simulink model "SegheriaSCADA2"  (R2024b)
settings: Solver=FixedStepAuto  StartTime=0.0  StopTime=2000  FixedStep=0.025  RelTol=1e-3
values from neighbouring files (symbols this model uses):
  b = t + 2*s    (= 3.6)    [ParametriSegheria.m]    (also in ParametriSegheriaDinamica.m; main_param_CLASSIC.m; main_param_SCADA.m)
  b2 = t2 + 2*s2    (= 10)    [ParametriSegheria.m]    (also in ParametriSegheriaDinamica.m; main_param_CLASSIC.m; main_param_SCADA.m)
  h_index = [70, 80, 90, 100]    [ParametriSegheria.m]    (also in ParametriSegheriaDinamica.m = [80, 90, 100]; main_param_CLASSIC.m = [80, 90, 100, 110]; main_param_SCADA.m = [80, 90, 100, 110])
  h_start_1 = 1    [main_param_CLASSIC.m]
  h_start_2 = 2    [main_param_CLASSIC.m]
  h_start_3 = 3    [main_param_CLASSIC.m]
  h_start_4 = 1    [main_param_CLASSIC.m]
  h_start_5 = 2    [main_param_CLASSIC.m]
  h_start_6 = 3    [main_param_CLASSIC.m]
  i_id = 60    [ParametriSegheria.m]
  i_id2 = 60    [ParametriSegheria.m]
  i_max = 100    [ParametriSegheria.m]
  kc = [0 35 40 50 55 90]    [ParametriSegheria.m]    (also in ParametriSegheriaDinamica.m = [0, 25, 30, 35, 50, 70]; main_param_CLASSIC.m = [0, 25, 30, 35, 50, 70]; main_param_SCADA.m = [0, 25, 30, 35, 50, 70])
  Kt = 2    [ParametriSegheria.m]    (also in ParametriSegheriaDinamica.m = 10000; main_param_CLASSIC.m = 10000; main_param_SCADA.m = 10000)
  Kt2 = 5    [ParametriSegheria.m]    (also in ParametriSegheriaDinamica.m = 4500; main_param_CLASSIC.m = 4500; main_param_SCADA.m = 4500)
  l_index = [20, 30, 40, 50]    [ParametriSegheria.m]    (also in ParametriSegheriaDinamica.m = [30, 40, 50]; main_param_CLASSIC.m = [30, 40, 50, 60]; main_param_SCADA.m = [30, 40, 50, 60])
  l_start_1 = 1    [main_param_CLASSIC.m]
  l_start_2 = 1    [main_param_CLASSIC.m]
  l_start_3 = 1    [main_param_CLASSIC.m]
  l_start_4 = 1    [main_param_CLASSIC.m]
  l_start_5 = 1    [main_param_CLASSIC.m]
  l_start_6 = 1    [main_param_CLASSIC.m]
  Lt = 4    [ParametriSegheria.m]    (also in ParametriSegheriaDinamica.m; main_param_CLASSIC.m; main_param_SCADA.m)
  Mag_D1 = [0 randi([220 500], 1, 40)]    [ParametriSegheria.m]    (also in ParametriSegheriaDinamica.m = [0 randi([200 500], 1, N_log)]; main_param_CLASSIC.m = [0 randi([200 500], 1, N_log)]; main_param_SCADA.m = [0 randi([200 500], 1, N_log)])
  Mag_D2 = [0 randi([220 500], 1, 40)]    [ParametriSegheria.m]    (also in ParametriSegheriaDinamica.m = [0 randi([200 500], 1, N_log)]; main_param_CLASSIC.m = [0 randi([200 500], 1, N_log)]; main_param_SCADA.m = [0 randi([200 500], 1, N_log)])
  Mag_D3 = [0 randi([220 500], 1, 40)]    [ParametriSegheria.m]    (also in ParametriSegheriaDinamica.m = [0 randi([200 500], 1, N_log)]; main_param_CLASSIC.m = [0 randi([200 500], 1, N_log)]; main_param_SCADA.m = [0 randi([200 500], 1, N_log)])
  Mag_legno1 = [0 randi([1 5], 1, 40)]    [ParametriSegheria.m]    (also in ParametriSegheriaDinamica.m = [0 randi([1 5], 1, N_log)]; main_param_CLASSIC.m = [0 randi([1 5], 1, N_log)]; main_param_SCADA.m = [0 randi([1 5], 1, N_log)])
  Mag_legno2 = [0 randi([1 5], 1, 40)]    [ParametriSegheria.m]    (also in ParametriSegheriaDinamica.m = [0 randi([1 5], 1, N_log)]; main_param_CLASSIC.m = [0 randi([1 5], 1, N_log)]; main_param_SCADA.m = [0 randi([1 5], 1, N_log)])
  Mag_legno3 = [0 randi([1 5], 1, 40)]    [ParametriSegheria.m]    (also in ParametriSegheriaDinamica.m = [0 randi([1 5], 1, N_log)]; main_param_CLASSIC.m = [0 randi([1 5], 1, N_log)]; main_param_SCADA.m = [0 randi([1 5], 1, N_log)])
  n_sottili = 4    [ParametriSegheria.m]
  omega = 50    [ParametriSegheria.m]
  omega2 = 3000*(2*pi/60)    (= 314.159265359)    [ParametriSegheria.m]
  SR = Rs/Rm    (= 5.33333333333)    [ParametriSegheria.m]    (also in ParametriSegheriaDinamica.m; main_param_CLASSIC.m; main_param_SCADA.m)
  SR2 = Rc/Rm2    (= 4)    [ParametriSegheria.m]    (also in ParametriSegheriaDinamica.m; main_param_CLASSIC.m; main_param_SCADA.m)
  thrsh = 40    [ParametriSegheria.m]
  Tloss = Tatt+ Tdamp    (= 17.3333333333)    [ParametriSegheria.m]
  Tloss2 = Tatt2+ Tdamp2    (= 66.8318530718)    [ParametriSegheria.m]
libraries: simulink x15, slpidlib x9
(part 3 of 3)

== matlab function SegheriaSCADA2/Linea 2/Macchina 2/MATLAB Function2 ==
  settings: updateMethod=DISCRETE
  data: u input; w_asse input; y output; l_asse input; taglio output; Lt parameter
function [y, taglio] = fcn(u, w_asse, l_asse,Lt)
    persistent counter 

    n_assi = floor(l_asse / w_asse);
    
    taglio = 0;

    if isempty(counter)
        counter = 0;
    end

    % Conto assi tagliate
    if u >= Lt
        counter = counter + n_assi;
    end

    % Segnale di taglio
    if  (u > 0 && u < Lt && l_asse > 0) 
        taglio = 1;
    end

    y = counter;
end

== matlab function SegheriaSCADA2/Linea 2/Macchina 3/MATLAB Function2 ==
  settings: updateMethod=DISCRETE
  data: u input; w_asse input; y output; l_asse input; taglio output; Lt parameter
function [y, taglio] = fcn(u, w_asse, l_asse,Lt)
    persistent counter 

    n_assi = floor(l_asse / w_asse);
    
    taglio = 0;

    if isempty(counter)
        counter = 0;
    end

    % Conto assi tagliate
    if u >= Lt
        counter = counter + n_assi;
    end

    % Segnale di taglio
    if  (u > 0 && u < Lt && l_asse > 0) 
        taglio = 1;
    end

    y = counter;
end

== matlab function SegheriaSCADA2/Linea 3/MATLAB Function ==
  data: u input; y output
function y = fcn(u)

    persistent n_prec

    if isempty(n_prec)
        n_prec = 0;
    end

    y = u - n_prec;


    n_prec = u;

== matlab function SegheriaSCADA2/Linea 3/MATLAB Function1 ==
  data: u input; y output
function y = fcn(u)

    persistent n_prec

    if isempty(n_prec)
        n_prec = 0;
    end

    y = u - n_prec;

    n_prec = u;

== matlab function SegheriaSCADA2/Linea 3/Macchina 1/Logica Macchina 1/MATLAB Function ==
  data: u input; y output; Mag_legno3 parameter
function y = fcn(u, Mag_legno3)
    persistent counter
    if isempty(counter)
        counter = 1;
    end

    if u == 1
        counter = counter + 1;
    end

    y = counter;
    
    if y > length(Mag_legno3)-1
        y = 0;
    end

end

== matlab function SegheriaSCADA2/Linea 3/Macchina 1/Logica Macchina 1/MATLAB Function2 ==
  settings: updateMethod=DISCRETE
  data: spessore input; u input; spessore2 input; thin_cut input; diametro input; y output; larg_asse output; thickness output; finito output
function [y, larg_asse, thickness, finito]= fcn(spessore, u, spessore2, thin_cut, diametro)
    persistent counter 

  
    max_assi = floor((diametro-thin_cut*spessore2) / spessore);
    finito = 0;
    
    if isempty(counter)
        counter = 0;
    end

    % Conto assi tagliate
    if u == 1
        counter = counter + 1;
    end

    % Quando finisco tronco segnalo e azzero counter
    if counter > max_assi + thin_cut
        finito = 1;
        counter = 0;
    end

    
    if counter == 0
        larg_asse = 0;
        thickness = 0;
    elseif counter <= thin_cut/2
        distanza_bordo = counter * spessore2;
        h = abs(diametro/2 - distanza_bordo + (spessore2/2));
        larg_asse = 2 * sqrt((diametro/2)^2-h^2);
        thickness = spessore2;
    elseif counter > max_assi + thin_cut/2
        distanza_bordo = max_assi*spessore + (counter-max_assi)*spessore2;
        h = abs(diametro/2 - distanza_bordo + (spessore2/2));
        larg_asse = 2 * sqrt((diametro/2)^2-h^2);
        thickness = spessore2;
    else
        % Calcolo larghezza delle assi
        distanza_bordo = thin_cut/2 * spessore2 + (counter-thin_cut/2) * spessore;
        h = abs(diametro/2 - distanza_bordo + (spessore/2));
        larg_asse = 2 * sqrt((diametro/2)^2-h^2);
        thickness = spessore;
    end
    

    y = counter;

== matlab function SegheriaSCADA2/Linea 1/Macchina 2/MATLAB Function2 ==
  settings: updateMethod=DISCRETE
  data: u input; w_asse input; y output; l_asse input; taglio output; Lt parameter
function [y, taglio] = fcn(u, w_asse, l_asse,Lt)
    persistent counter 

    n_assi = floor(l_asse / w_asse);
    
    taglio = 0;

    if isempty(counter)
        counter = 0;
    end

    % Conto assi tagliate
    if u >= Lt
        counter = counter + n_assi;
    end

    % Segnale di taglio
    if  (u > 0 && u < Lt && l_asse > 0) 
        taglio = 1;
    end

    y = counter;
end

== matlab function SegheriaSCADA2/Linea 3/Macchina 2/MATLAB Function2 ==
  settings: updateMethod=DISCRETE
  data: u input; w_asse input; y output; l_asse input; taglio output; Lt parameter
function [y, taglio] = fcn(u, w_asse, l_asse,Lt)
    persistent counter 

    n_assi = floor(l_asse / w_asse);
    
    taglio = 0;

    if isempty(counter)
        counter = 0;
    end

    % Conto assi tagliate
    if u >= Lt
        counter = counter + n_assi;
    end

    % Segnale di taglio
    if  (u > 0 && u < Lt && l_asse > 0) 
        taglio = 1;
    end

    y = counter;
end

== matlab function SegheriaSCADA2/Linea 3/Macchina 3/MATLAB Function2 ==
  settings: updateMethod=DISCRETE
  data: u input; w_asse input; y output; l_asse input; taglio output; Lt parameter
function [y, taglio] = fcn(u, w_asse, l_asse,Lt)
    persistent counter 

    n_assi = floor(l_asse / w_asse);
    
    taglio = 0;

    if isempty(counter)
        counter = 0;
    end

    % Conto assi tagliate
    if u >= Lt
        counter = counter + n_assi;
    end

    % Segnale di taglio
    if  (u > 0 && u < Lt && l_asse > 0) 
        taglio = 1;
    end

    y = counter;
end

== matlab function SegheriaSCADA2/Subsystem1/MATLAB Function6 ==
  data: u input; idx output; h_index parameter
function idx = find_index(u, h_index)
%#codegen

v = h_index;

idx = -1; % valore default se non trovato

for i = 1:length(v)
    if u == v(i)
        idx = i;
        return;
    end
end

== matlab function SegheriaSCADA2/Subsystem1/MATLAB Function7 ==
  data: u input; idx output; h_index parameter
function idx = find_index(u, h_index)
%#codegen

v = h_index;

idx = -1; % valore default se non trovato

for i = 1:length(v)
    if u == v(i)
        idx = i;
        return;
    end
end

== matlab function SegheriaSCADA2/Subsystem1/MATLAB Function8 ==
  data: u input; idx output; h_index parameter
function idx = find_index(u, h_index)
%#codegen

v = h_index;

idx = -1; % valore default se non trovato

for i = 1:length(v)
    if u == v(i)
        idx = i;
        return;
    end
end

== matlab function SegheriaSCADA2/Subsystem1/MATLAB Function9 ==
  data: u input; idx output; h_index parameter
function idx = find_index(u, h_index)
%#codegen

v = h_index;

idx = -1; % valore default se non trovato

for i = 1:length(v)
    if u == v(i)
        idx = i;
        return;
    end
end

== matlab function SegheriaSCADA2/Subsystem1/MATLAB Function10 ==
  data: u input; idx output; l_index parameter
function idx = find_index(u, l_index)
%#codegen

v = l_index;

idx = -1; % valore default se non trovato

for i = 1:length(v)
    if u == v(i)
        idx = i;
        return;
    end
end

== matlab function SegheriaSCADA2/Subsystem1/MATLAB Function11 ==
  data: u input; idx output; l_index parameter
function idx = find_index(u, l_index)
%#codegen

v = l_index;

idx = -1; % valore default se non trovato

for i = 1:length(v)
    if u == v(i)
        idx = i;
        return;
    end
end

== matlab function SegheriaSCADA2/Subsystem1/MATLAB Function12 ==
  data: u input; idx output; l_index parameter
function idx = find_index(u, l_index)
%#codegen

v = l_index;

idx = -1; % valore default se non trovato

for i = 1:length(v)
    if u == v(i)
        idx = i;
        return;
    end
end

== matlab function SegheriaSCADA2/Subsystem1/MATLAB Function13 ==
  data: u input; idx output; l_index parameter
function idx = find_index(u, l_index)
%#codegen

v = l_index;

idx = -1; % valore default se non trovato

for i = 1:length(v)
    if u == v(i)
        idx = i;
        return;
    end
end

== matlab function SegheriaSCADA2/Subsystem1/MATLAB Function14 ==
  data: h_next output; Magazzino output; work output; l_next output; h_idx input; target_matrice parameter; n_assi input; l_idx input
function [h_next, Magazzino, work, l_next] = fcn(h_idx, target_matrice, n_assi, l_idx)

[n_rows, n_cols] = size(target_matrice);

h_next = zeros(1,length(h_idx));
l_next = zeros(1,length(l_idx));

persistent MagazzinoGlobale

for i = 1:length(n_assi)

    if isempty(MagazzinoGlobale)
        MagazzinoGlobale = zeros(n_rows, n_cols);
    end


    % Output iniziali
    h_next(i) = h_idx(i);
    l_next(i) = l_idx(i);


    MagazzinoGlobale(h_idx(i), l_idx(i)) = MagazzinoGlobale(h_idx(i), l_idx(i)) + n_assi(i);

    work = 1;

    if MagazzinoGlobale(h_idx(i), l_idx(i)) >= target_matrice(h_idx(i), l_idx(i))


        deficit = target_matrice - MagazzinoGlobale;

        best_cost = inf;
        best_h = h_idx(i);
        best_l = l_idx(i);

        for h = 1:n_rows
            for l = 1:n_cols

                if deficit(h,l) > 0

                    % Penalità cambio lama
                    cambio = (l ~= l_idx(i));

                    % Funzione costo
                    cost = -deficit(h,l) + 60*cambio;

                    if cost < best_cost
                        best_cost = cost;
                        best_h = h;
                        best_l = l;
                    end
                end

            end
        end

        if best_cost < inf
            h_next(i) = best_h;
            l_next(i) = best_l;
        else
            work = 0;
        end

    end
end

Magazzino = MagazzinoGlobale;

== matlab function SegheriaSCADA2/Linea 1/Macchina 1/Dinamica Macchina 1/MATLAB Function ==
  settings: updateMethod=DISCRETE
  data: u input; y output; t input
function y = f(u, t)
persistent t_start active

if isempty(active)
    active = false;
    t_start = 0;
end

if u == 1 && ~active
    t_start = t;
    active = true;
end

if active
    if (t - t_start) <= 180
        y = 0;
    else
        y = 1;
        active = false;
    end
else
    y = 1;
end

== matlab function SegheriaSCADA2/Subsystem1/CAMBIO LAME CONSUMATE ==
  data: n_assi input; y output; cambio_1 output; cambio_2 output; cambio_3 output
function [y, cambio_1, cambio_2, cambio_3] = fcn(n_assi)

    warning = zeros(1, length(n_assi));

    persistent usura_lama

    if isempty(usura_lama)
        usura_lama = zeros(1, length(n_assi));
    end

    cambio_1 = 0;
    cambio_2 = 0;
    cambio_3 = 0;

    for i = 1:length(n_assi)
        
        % Ogni volta che arriva un certo numero di assi vuol dire che le
        % lame hanno appena fatto un taglio
        if n_assi(i) ~= 0
            usura_lama(i) = usura_lama(i) + 1;
        end
        
        if 20 - usura_lama(i) < 2
            warning(i) = 1;
            usura_lama(i) = 0;
        end

        % i = 1 -> M2 Linea 1
        % i = 2 -> M3 Linea 1
        % i = 3 -> M2 Linea 2
        % i = 4 -> M3 Linea 2
        % i = 5 -> M2 Linea 3
        % i = 6 -> M2 Linea 3
        if (i == 1 || i == 2) && warning(i) == 1
            cambio_1 = 1;
        elseif (i == 3 || i == 4) && warning(i) == 1
            cambio_2 = 1;
        elseif (i == 5 || i == 6) && warning(i) == 1
            cambio_3 = 1;
        end

    end

    y = warning;

== matlab function SegheriaSCADA2/Linea 1/Macchina 1/Logica Macchina 1/MATLAB Function ==
  data: u input; y output; Mag_legno1 parameter
function y = fcn(u, Mag_legno1)
    persistent counter
    if isempty(counter)
        counter = 1;
    end

    if u == 1
        counter = counter + 1;
    end

    y = counter;
    
    if y > length(Mag_legno1)-1
        y = 0;
    end

end

== matlab function SegheriaSCADA2/Linea 2/Macchina 1/Dinamica Macchina 1/MATLAB Function ==
  settings: updateMethod=DISCRETE
  data: u input; y output; t input
function y = f(u, t)
persistent t_start active

if isempty(active)
    active = false;
    t_start = 0;
end

if u == 1 && ~active
    t_start = t;
    active = true;
end

if active
    if (t - t_start) <= 180
        y = 0;
    else
        y = 1;
        active = false;
    end
else
    y = 1;
end

== matlab function SegheriaSCADA2/Linea 3/Macchina 1/Dinamica Macchina 1/MATLAB Function ==
  settings: updateMethod=DISCRETE
  data: u input; y output; t input
function y = f(u, t)
persistent t_start active

if isempty(active)
    active = false;
    t_start = 0;
end

if u == 1 && ~active
    t_start = t;
    active = true;
end

if active
    if (t - t_start) <= 180
        y = 0;
    else
        y = 1;
        active = false;
    end
else
    y = 1;
end

== matlab function SegheriaSCADA2/Linea 1/Macchina 1/Dinamica Macchina 1/MATLAB Function1 ==
  data: lama_usurata input; y output; tronco_finito input
function y = fcn(lama_usurata, tronco_finito)
    
    persistent cambia_lama
    if isempty(cambia_lama)
        cambia_lama = 0;
    end

    if lama_usurata == 1
        cambia_lama = 1;
    end

    if tronco_finito == 1 && cambia_lama == 1
        y = cambia_lama;
        cambia_lama = 0;
    else
        y = 0;
    end

== matlab function SegheriaSCADA2/Linea 2/Macchina 1/Dinamica Macchina 1/MATLAB Function1 ==
  data: lama_usurata input; y output; tronco_finito input
function y = fcn(lama_usurata, tronco_finito)
    
    persistent cambia_lama
    if isempty(cambia_lama)
        cambia_lama = 0;
    end

    if lama_usurata == 1
        cambia_lama = 1;
    end

    if tronco_finito == 1 && cambia_lama == 1
        y = cambia_lama;
        cambia_lama = 0;
    else
        y = 0;
    end

== matlab function SegheriaSCADA2/Linea 3/Macchina 1/Dinamica Macchina 1/MATLAB Function1 ==
  data: lama_usurata input; y output; tronco_finito input
function y = fcn(lama_usurata, tronco_finito)
    
    persistent cambia_lama
    if isempty(cambia_lama)
        cambia_lama = 0;
    end

    if lama_usurata == 1
        cambia_lama = 1;
    end

    if tronco_finito == 1 && cambia_lama == 1
        y = cambia_lama;
        cambia_lama = 0;
    else
        y = 0;
    end

== matlab function SegheriaSCADA2/Linea 1/Macchina 1/Logica Macchina 1/MATLAB Function2 ==
  settings: updateMethod=DISCRETE
  data: spessore input; u input; spessore2 input; thin_cut input; diametro input; y output; larg_asse output; thickness output; finito output
function [y, larg_asse, thickness, finito]= fcn(spessore, u, spessore2, thin_cut, diametro)
    persistent counter 

  
    max_assi = floor((diametro-thin_cut*spessore2) / spessore);
    finito = 0;
    
    if isempty(counter)
        counter = 0;
    end

    % Conto assi tagliate
    if u == 1
        counter = counter + 1;
    end

    % Quando finisco tronco segnalo e azzero counter
    if counter > max_assi + thin_cut
        finito = 1;
        counter = 0;
    end

    
    if counter == 0
        larg_asse = 0;
        thickness = 0;
    elseif counter <= thin_cut/2
        distanza_bordo = counter * spessore2;
        h = abs(diametro/2 - distanza_bordo + (spessore2/2));
        larg_asse = 2 * sqrt((diametro/2)^2-h^2);
        thickness = spessore2;
    elseif counter > max_assi + thin_cut/2
        distanza_bordo = max_assi*spessore + (counter-max_assi)*spessore2;
        h = abs(diametro/2 - distanza_bordo + (spessore2/2));
        larg_asse = 2 * sqrt((diametro/2)^2-h^2);
        thickness = spessore2;
    else
        % Calcolo larghezza delle assi
        distanza_bordo = thin_cut/2 * spessore2 + (counter-thin_cut/2) * spessore;
        h = abs(diametro/2 - distanza_bordo + (spessore/2));
        larg_asse = 2 * sqrt((diametro/2)^2-h^2);
        thickness = spessore;
    end
    

    y = counter;

== matlab function SegheriaSCADA2/Linea 1/Macchina 3/MATLAB Function2 ==
  settings: updateMethod=DISCRETE
  data: u input; w_asse input; y output; l_asse input; taglio output; Lt parameter
function [y, taglio] = fcn(u, w_asse, l_asse,Lt)
    persistent counter 

    n_assi = floor(l_asse / w_asse);
    
    taglio = 0;

    if isempty(counter)
        counter = 0;
    end

    % Conto assi tagliate
    if u >= Lt
        counter = counter + n_assi;
    end

    % Segnale di taglio
    if  (u > 0 && u < Lt && l_asse > 0) 
        taglio = 1;
    end

    y = counter;
end

== matlab function SegheriaSCADA2/Linea 1/MATLAB Function ==
  data: u input; y output
function y = fcn(u)

    persistent n_prec

    if isempty(n_prec)
        n_prec = 0;
    end

    y = u - n_prec;


    n_prec = u;

== matlab function SegheriaSCADA2/Subsystem1/MATLAB Function1 ==
  data: u input; idx output; h_index parameter
function idx = find_index(u, h_index)
%#codegen

v = h_index;

idx = -1; % valore default se non trovato

for i = 1:length(v)
    if u == v(i)
        idx = i;
        return;
    end
end

== matlab function SegheriaSCADA2/Subsystem1/MATLAB Function2 ==
  data: u input; idx output; l_index parameter
function idx = find_index(u, l_index)
%#codegen

v = l_index;

idx = -1; % valore default se non trovato

for i = 1:length(v)
    if u == v(i)
        idx = i;
        return;
    end
end

== matlab function SegheriaSCADA2/Subsystem1/MATLAB Function3 ==
  data: h_next output; Magazzino output; work output; l_next output; h_idx input; target_matrice parameter; n_assi input; l_idx input; cambio_lama_idx output
function [h_next, Magazzino, work, l_next, cambio_lama_idx] = fcn(h_idx, target_matrice, n_assi, l_idx)

[n_rows, n_cols] = size(target_matrice);

h_next = zeros(1,length(h_idx));
l_next = zeros(1,length(l_idx));

persistent MagazzinoReale
persistent x_hat
persistent P

persistent usura_lama

if isempty(MagazzinoReale)
    MagazzinoReale = zeros(n_rows, n_cols);
    x_hat = zeros(n_rows, n_cols);
    P = eye(n_rows*n_cols);
    usura_lama = zeros(1, length(n_assi));
end

cambio_lama_idx = zeros(1, length(n_assi));
for i = 1:length(n_assi)

    % Output iniziali
    h_next(i) = h_idx(i);
    l_next(i) = l_idx(i);

    MagazzinoReale(h_idx(i), l_idx(i)) = MagazzinoReale(h_idx(i), l_idx(i)) + n_assi(i);

end






work = 1;
    
% MISURA RUMOROSA
sigma = 0.1;
y = MagazzinoReale + sigma*randn(size(MagazzinoReale));


% APPIATTISCO MATRICE
x_hat_vec = x_hat(:);
y_vec = y(:);
u = zeros(size(x_hat_vec));

% PREDICTION
Q = 0.01*eye(length(x_hat_vec));
x_pred = x_hat_vec + u;
P_pred = P + Q;

% UPDATE
R = 1*eye(length(x_hat_vec));
K = P_pred / (P_pred + R);
x_hat_vec = x_pred + K*(y_vec - x_pred);
P = (eye(size(K)) - K)*P_pred;

x_hat = reshape(x_hat_vec, n_rows, n_cols);


for i = 1:length(n_assi)
    if MagazzinoReale(h_idx(i), l_idx(i)) >= target_matrice(h_idx(i), l_idx(i))


        deficit = target_matrice - MagazzinoReale;

        best_cost = inf;
        best_h = h_idx(i);
        best_l = l_idx(i);

        for h = 1:n_rows
            for l = 1:n_cols

                if deficit(h,l) > 0

                    % Penalità cambio lama
                    cambio = (l ~= l_idx(i));

                    % Funzione costo
                    cost = -deficit(h,l) + 60*cambio;

                    if cost < best_cost
                        best_cost = cost;
                        best_h = h;
                        best_l = l;
                    end
                end

            end
        end

        if best_cost < inf
            h_next(i) = best_h;
            l_next(i) = best_l;
        else
            work = 0;
        end

    end
end

Magazzino = MagazzinoReale;
